simulink model "mod_adcs3"  (R2016a)
settings: Solver=ode45  SolverMode=SingleTasking  StartTime=0.0  StopTime=500  RelTol=1e-3
values from neighbouring files (symbols this model uses):
  A = E*G'    [angls.m]
libraries: vrlib x1
settings Model: Creator=Mohammed Hussein  LastModifiedBy=M
settings DataIOCC: SaveFormat=StructureWithTime
settings DebuggingCC: SFUnexpectedBacktrackingDiag=error  SFNoUnconditionalDefaultTransitionDiag=error
settings HardwareCC: ProdWordSize=32  ProdHWDeviceType=Specified
settings GRTTargetCC: TargetLangStandard=C99 (ISO)  GeneratePreprocessorConditionals=Use local settings
settings ConfigComp: CovMetricSettings=dwe  CovHtmlReporting=off  CovSaveCumulativeToWorkspaceVar=off  CovSaveSingleToWorkspaceVar=off  CovModelRefEnable=Off  CovExternalEMLEnable=on

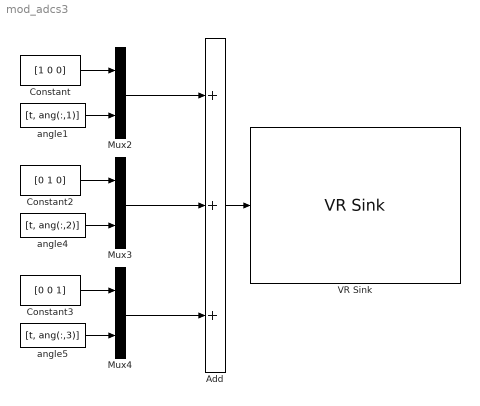
== system mod_adcs3 ==
  Add : Sum  Inputs=+++
  Constant : Constant  Value=[1 0 0]
  Constant2 : Constant  Value=[0 1 0]
  Constant3 : Constant  Value=[0 0 1]
  Mux2 : Mux  Inputs=2
  Mux3 : Mux  Inputs=2
  Mux4 : Mux  Inputs=2
  VR Sink : vrlib/VR Sink  InstantiateOnLoad=on  SampleTime=0.1  ViewEnable=on  RemoteChange=off  RemoteView=off  FieldsWritten=Box.rotation.4.1.1.double  WorldFileName=E:\A\ADC\project\satell.wrl  AutoView=off  VideoDimensions=[]  AllowVariableSize=off  FigureProperties="{'Position', 'Name', 'Viewpoint', 'CameraBound', 'CameraDirection', 'CameraPosition', 'CameraUpVector', 'ZoomFactor', 'Antialiasing', 'Headlight', 'Lighting', 'NavPanel', 'Sound', 'StatusBar', 'Stereo3D', 'Stereo3DCameraOffset', 'Stereo3DHIT', 'ToolBar', 'Textures', 'Transparency', 'Triad', 'Wireframe', 'NavZones', 'NavMode', 'NavSpeed', 'CaptureFileFormat', 'CaptureFileName', 'Record2DCompressMethod', 'Record2DCompressQuality', 'Record2D', 'Record2DFileName', 'Record2DFPS'; [1.0000000000000000e+00   7.5000000000000000e+01   1.2800000000000000e+03   6.4400000000000000e+02], '', '', 'on', [5.8260253968086062e-01   7.9482255803675039e-01   1.6979806239583883e-01], [-5.8260253968086202e+00  -7.9482255803674979e+00  -1.6979806239584110e+00], [1.0661688802262007e-01   1.3237184709763225e-01  -9.8544940676036752e-01], [1.0000000000000000e+00], 'on', 'on', 'on', 'halfbar', 'on', 'on', 'off', [1.0000000149011612e-01], [0.0000000000000000e+00], 'on', 'on', 'on', 'none', 'off', 'off', 'examine', 'normal', 'tif', '%f_anim_%n.tif', 'auto', [7.5000000000000000e+01], 'off', '%f_anim_%n.avi', 'auto'}"
  angle1 : FromWorkspace  VariableName=[t, ang(:,1)]  SampleTime=0
  angle4 : FromWorkspace  VariableName=[t, ang(:,2)]  SampleTime=0
  angle5 : FromWorkspace  VariableName=[t, ang(:,3)]  SampleTime=0
  wires:
  Constant/1 -> Mux2/1
  angle1/1 -> Mux2/2
  Add/1 -> VR Sink/1
  Mux2/1 -> Add/1
  Constant2/1 -> Mux3/1
  angle4/1 -> Mux3/2
  Mux3/1 -> Add/2
  Constant3/1 -> Mux4/1
  angle5/1 -> Mux4/2
  Mux4/1 -> Add/3
